simulink model "test1_2"  (R2018b)
settings: Solver=VariableStepAuto  StartTime=0.0  StopTime=1.0  RelTol=1e-3
libraries: commchan3 x1, dsparch4 x1
settings Model: Creator=Aurora  LastModifiedBy=Aurora

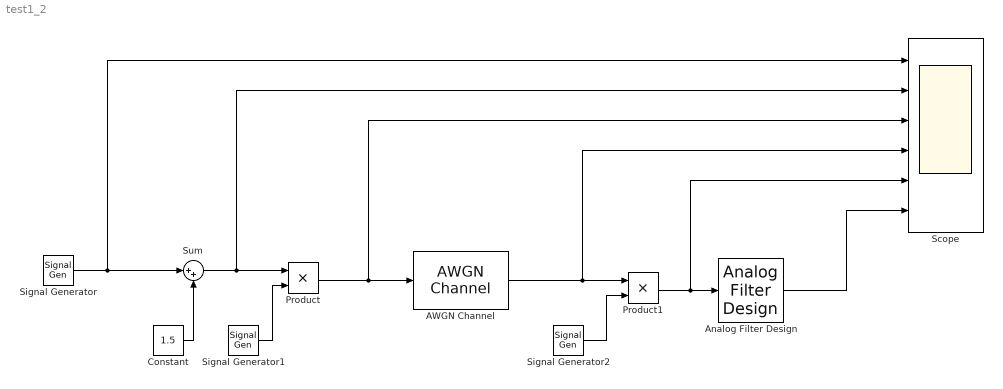
== system test1_2 ==
  AWGN Channel : commchan3/AWGN Channel  InputProcessing=Columns as channels (frame based)  seed=67  noiseMode="Signal to noise ratio  (SNR)"  EbNodB=10  EsNodB=10  SNRdB=10  bitsPerSym=1  Ps=1  Tsym=1  variance=1
  Analog Filter Design : dsparch4/Analog Filter Design  method=Butterworth  filttype=Lowpass  N=8  Wlo=2*pi*3000  Whi=80  Rp=2  Rs=40
  Constant : Constant  Value=1.5
  Product : Product
  Product1 : Product
  Scope : Scope  NumInputPorts=6
  Signal Generator : SignalGenerator  Frequency=3000
  Signal Generator1 : SignalGenerator  Frequency=90000
  Signal Generator2 : SignalGenerator  Frequency=90000
  Sum : Sum  Inputs=|++
  wires:
  AWGN Channel/1 -> Scope/4, Product1/1
  Signal Generator/1 -> Scope/1, Sum/1
  Product1/1 -> Analog Filter Design/1, Scope/5
  Analog Filter Design/1 -> Scope/6
  Product/1 -> Scope/3, AWGN Channel/1
  Signal Generator2/1 -> Product1/2
  Constant/1 -> Sum/2
  Signal Generator1/1 -> Product/2
  Sum/1 -> Scope/2, Product/1
